simulink model "Boat_mode"  (R2019a)
settings: Solver=VariableStepAuto  StartTime=0.0  StopTime=3000  RelTol=1e-3
InitFcn:
  | w = 0.3;
  | boat_m = 600;
  | boat_m_x = 50;
  | boat_m_y = 100;
  | 
  | boat_I = 6000000;
  | boat_Iz = 10;
  | 
  | propeller_diameter = 1;
  | wake_friction=0.3;
  | 
  | c_r_front = 0.31;
  | c_r_side = 2;
  | thrust_deduction = 0.3;
  | 
  | rho = 1;
  | 
  | boat_area_front = 20;
  | boat_area_side = 90;
  | boat_l = 15;
  | boat_b = 6;
  | 
  | rudder_area = 10;
  | aspect_ratio = 2;
  | a = 4.252;
  | b = 0.262;
  | 
  | plot =20000;
libraries: simulink x7, simulink_extras x3
settings Model: Creator=nicos  LastModifiedBy=nicos
settings DataIOCC: SaveState=on

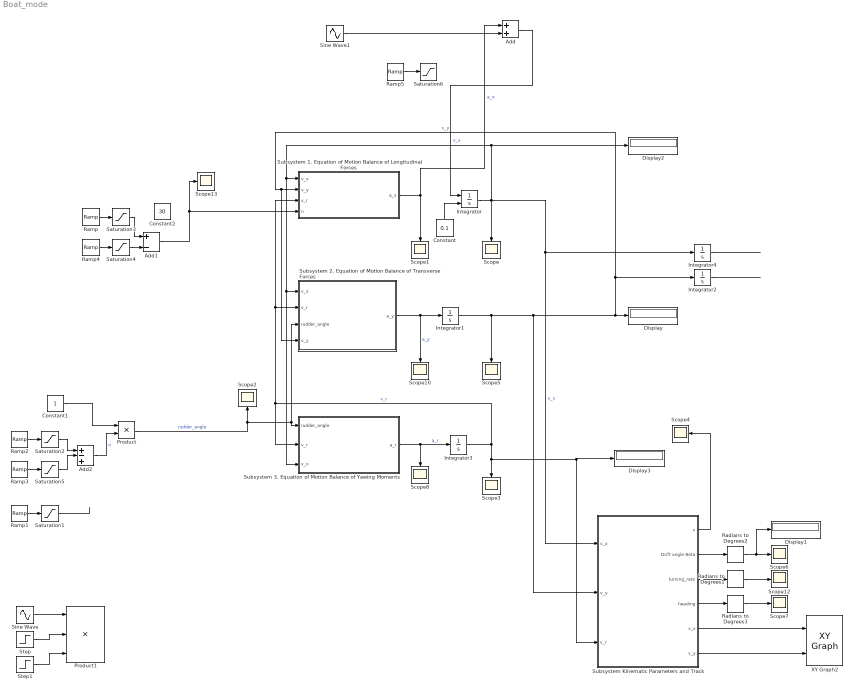
== system Boat_mode ==
  Add : Sum
  Add1 : Sum  Inputs=+-
  Add2 : Sum  Inputs=+-+
  Constant : Constant  Value=0.1
  Constant1 : Constant
  Constant2 : Constant  Value=30
  Display{,1..3} (4 alike) : Display
  Integrator : Integrator  InitialConditionSource=external  LimitOutput=on  LowerSaturationLimit=0
  Integrator{1..4} (4 alike) : Integrator
  Product : Product
  Product1 : Product  Inputs=3
  Radians to Degrees1 : simulink_extras/Transformations/Radians to Degrees
  Radians to Degrees2 : simulink_extras/Transformations/Radians to Degrees
  Radians to Degrees3 : simulink_extras/Transformations/Radians to Degrees
  Ramp : simulink/Sources/Ramp  slope=2  start=50  InitialOutput=0
  Ramp1 : simulink/Sources/Ramp  slope=0.01  start=1500  InitialOutput=0
  Ramp2 : simulink/Sources/Ramp  slope=0.01  start=500  InitialOutput=0
  Ramp3 : simulink/Sources/Ramp  slope=0.01  start=1000  InitialOutput=0
  Ramp4 : simulink/Sources/Ramp  slope=0.1  start=1300  InitialOutput=0
  Ramp5 : simulink/Sources/Ramp  slope=0.1  start=500  InitialOutput=0
  Saturation1 : Saturate  UpperLimit=pi/4  LowerLimit=0
  Saturation2 : Saturate  UpperLimit=pi/4  LowerLimit=0
  Saturation3 : Saturate  UpperLimit=20  LowerLimit=0
  Saturation4 : Saturate  UpperLimit=20  LowerLimit=0
  Saturation5 : Saturate  UpperLimit=pi/2  LowerLimit=0
  Saturation6 : Saturate  UpperLimit=1  LowerLimit=0
  Scope{,1..8,10,12..13} (12 alike) : Scope
  Sine Wave : Sin  Amplitude=pi/4  Frequency=0.01  SampleTime=0
  Sine Wave1 : Sin  Amplitude=0  Frequency=0.005  SampleTime=0
  Step : Step  Time=0  SampleTime=0
  Step1 : Step  Time=2000  Before=1  After=0  SampleTime=0
  Subsystem Kinematic Parameters and Track : Subsystem
  Subsystem 1. Equation of Motion Balance of Longitudinal Forces : Subsystem
  Subsystem 2. Equation of Motion Balance of Transverse Forces : Subsystem
  Subsystem 3. Equation of Motion Balance of Yawing Moments : Subsystem
  XY Graph2 : simulink/Sinks/XY Graph  xmin=-plot  xmax=plot  ymin=-plot  ymax=plot  st=-1
  wires:
  Subsystem 1. Equation of Motion Balance of Longitudinal Forces/1(a_x) -> Add/1, Scope1/1  "a_x"
  Constant/1 -> Integrator/2
  Integrator/1 -> Subsystem 2. Equation of Motion Balance of Transverse Forces/1(v_x), Subsystem 3. Equation of Motion Balance of Yawing Moments/3(v_x), Subsystem 1. Equation of Motion Balance of Longitudinal Forces/1(v_x), Display2/1, Integrator4/1, Subsystem Kinematic Parameters and Track/1(v_x), Scope/1  "v_x"
  Subsystem 3. Equation of Motion Balance of Yawing Moments/1(a_r) -> Integrator3/1, Scope8/1  "a_r"
  Subsystem 2. Equation of Motion Balance of Transverse Forces/1(a_y) -> Integrator1/1, Scope10/1  "a_y"
  Subsystem Kinematic Parameters and Track/1(v) -> Scope4/1
  Subsystem Kinematic Parameters and Track/5(s_x) -> XY Graph2/1
  Subsystem Kinematic Parameters and Track/6(s_y) -> XY Graph2/2
  Ramp4/1 -> Saturation4/1
  Saturation3/1 -> Add1/1
  Saturation4/1 -> Add1/2
  Ramp/1 -> Saturation3/1
  Subsystem Kinematic Parameters and Track/2(Drift angle Beta) -> Radians to Degrees2/1
  Subsystem Kinematic Parameters and Track/3(turning_rate) -> Radians to Degrees1/1
  Radians to Degrees1/1 -> Scope12/1
  Radians to Degrees2/1 -> Display1/1, Scope6/1
  Subsystem Kinematic Parameters and Track/4(heading) -> Radians to Degrees3/1
  Radians to Degrees3/1 -> Scope7/1
  Integrator3/1 -> Subsystem 2. Equation of Motion Balance of Transverse Forces/2(v_r), Subsystem 1. Equation of Motion Balance of Longitudinal Forces/3(v_r), Subsystem 3. Equation of Motion Balance of Yawing Moments/2(v_r), Display3/1, Subsystem Kinematic Parameters and Track/3(v_r), Scope3/1  "v_r"
  Product/1 -> Scope2/1, Subsystem 2. Equation of Motion Balance of Transverse Forces/3(rudder_angle), Subsystem 3. Equation of Motion Balance of Yawing Moments/1(rudder_angle)  "rudder_angle"
  Constant1/1 -> Product/1
  Integrator4/1 -> ?
  Integrator2/1 -> ?
  Saturation2/1 -> Add2/1
  Ramp3/1 -> Saturation5/1
  Saturation5/1 -> Add2/2
  Ramp2/1 -> Saturation2/1
  Add2/1 -> Product/2  "n"
  Add1/1 -> Subsystem 1. Equation of Motion Balance of Longitudinal Forces/4(n), Scope13/1
  Ramp1/1 -> Saturation1/1
  Saturation1/1 -> ?
  Sine Wave/1 -> Product1/1
  Step/1 -> Product1/2
  Step1/1 -> Product1/3
  Integrator1/1 -> Scope5/1, Subsystem Kinematic Parameters and Track/2(v_y), Display/1, Integrator2/1, Subsystem 2. Equation of Motion Balance of Transverse Forces/4(v_y), Subsystem 1. Equation of Motion Balance of Longitudinal Forces/2(v_y)  "v_y"
  Sine Wave1/1 -> Add/2
  Ramp5/1 -> Saturation6/1
  Add/1 -> Integrator/1  "v_x"

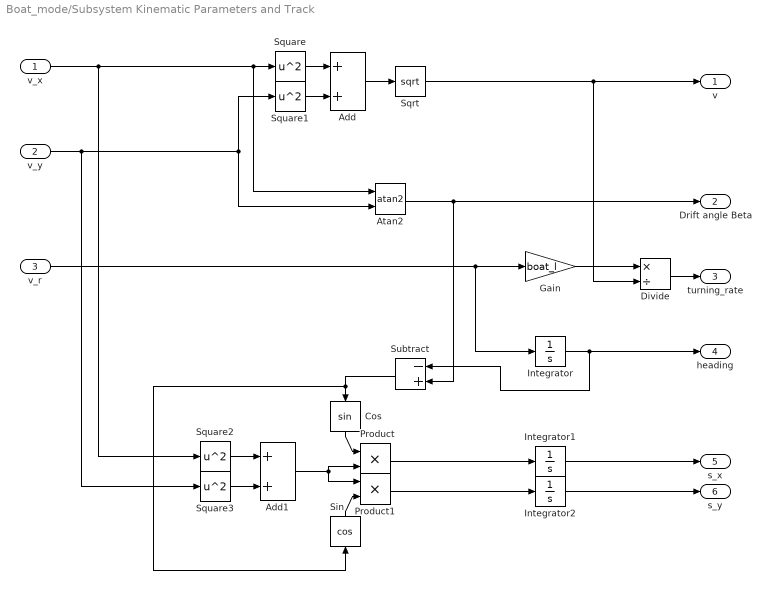
== system Boat_mode/Subsystem Kinematic Parameters and Track ==
  v_x : Inport
  v_y : Inport  Port=2
  v_r : Inport  Port=3
  Add : Sum
  Add1 : Sum
  Atan2 : Trigonometry  Operator=atan2
  Cos : Trigonometry
  Divide : Product  Inputs=*/
  Gain : Gain  Gain=boat_l
  Integrator : Integrator
  Integrator1 : Integrator
  Integrator2 : Integrator
  Product : Product
  Product1 : Product
  Sin : Trigonometry  Operator=cos
  Sqrt : Sqrt  SaturateOnIntegerOverflow=on
  Square{,1..3} (4 alike) : Math  Operator=square  SaturateOnIntegerOverflow=on
  Subtract : Sum  Inputs=-+
  v : Outport
  Drift angle Beta : Outport  Port=2
  turning_rate : Outport  Port=3
  heading : Outport  Port=4
  s_x : Outport  Port=5
  s_y : Outport  Port=6
  wires:
  v_x/1 -> Square2/1, Atan2/1, Square/1
  v_y/1 -> Square3/1, Atan2/2, Square1/1
  Square/1 -> Add/1
  Square1/1 -> Add/2
  Add/1 -> Sqrt/1
  Sqrt/1 -> v/1, Divide/2
  Gain/1 -> Divide/1
  Divide/1 -> turning_rate/1
  v_r/1 -> Integrator/1, Gain/1
  Integrator/1 -> Subtract/1, heading/1
  Integrator1/1 -> s_x/1
  Integrator2/1 -> s_y/1
  Atan2/1 -> Subtract/2, Drift angle Beta/1
  Square2/1 -> Add1/1
  Square3/1 -> Add1/2
  Add1/1 -> Product1/1, Product/2
  Subtract/1 -> Sin/1, Cos/1
  Cos/1 -> Product/1
  Product/1 -> Integrator1/1
  Product1/1 -> Integrator2/1
  Sin/1 -> Product1/2

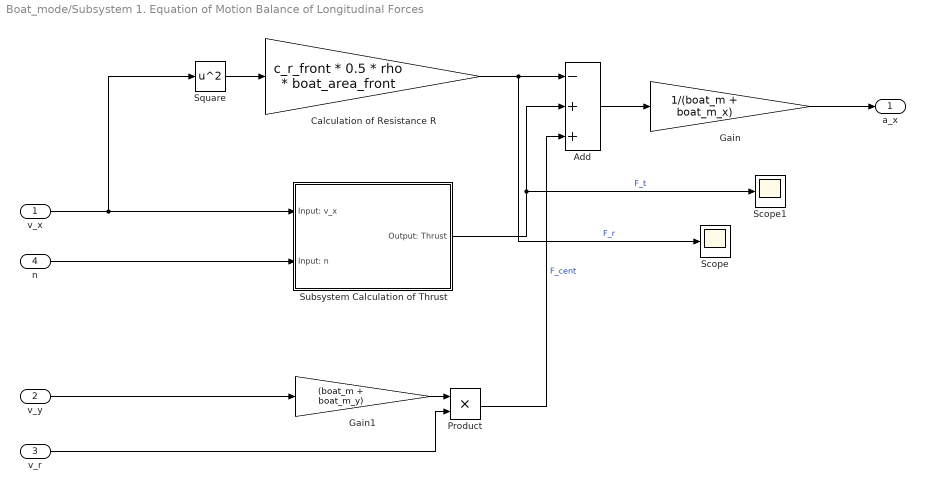
== system Boat_mode/Subsystem 1. Equation of Motion Balance of Longitudinal Forces ==
  v_x : Inport
  v_y : Inport  Port=2
  v_r : Inport  Port=3
  n : Inport  Port=4
  Add : Sum  Inputs=-++
  Calculation of Resistance R : Gain  Gain=c_r_front * 0.5 * rho * boat_area_front
  Gain : Gain  Gain=1/(boat_m + boat_m_x)
  Gain1 : Gain  Gain=(boat_m + boat_m_y)
  Product : Product
  Scope : Scope
  Scope1 : Scope
  Square : Math  Operator=square  SaturateOnIntegerOverflow=on
  Subsystem Calculation of Thrust : Subsystem
  a_x : Outport
  wires:
  v_x/1 -> Square/1, Subsystem Calculation of Thrust/1(Input: v_x)
  n/1 -> Subsystem Calculation of Thrust/2(Input: n)
  Square/1 -> Calculation of Resistance R/1
  Calculation of Resistance R/1 -> Scope/1, Add/1  "F_r"
  Subsystem Calculation of Thrust/1(Output: Thrust) -> Scope1/1, Add/2  "F_t"
  Add/1 -> Gain/1
  Gain/1 -> a_x/1
  v_y/1 -> Gain1/1
  Gain1/1 -> Product/1
  v_r/1 -> Product/2
  Product/1 -> Add/3  "F_cent"

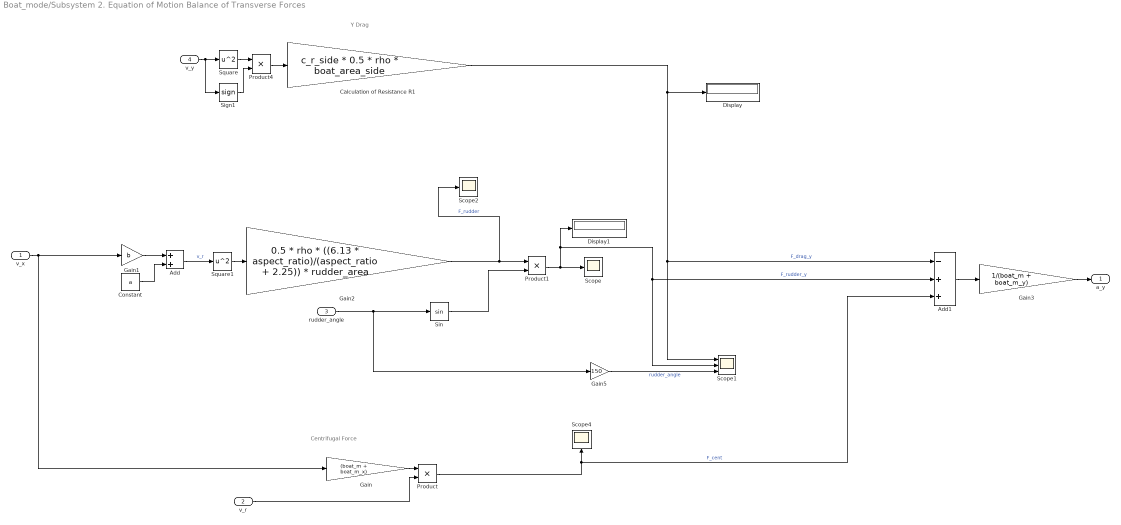
== system Boat_mode/Subsystem 2. Equation of Motion Balance of Transverse Forces ==
  note: Y Drag
  note: Centrifugal Force
  v_x : Inport
  v_r : Inport  Port=2
  rudder_angle : Inport  Port=3
  v_y : Inport  Port=4
  Add : Sum
  Add1 : Sum  Inputs=-++
  Calculation of Resistance R1 : Gain  Gain=c_r_side * 0.5 * rho * boat_area_side
  Constant : Constant  Value=a
  Display : Display
  Display1 : Display
  Gain : Gain  Gain=(boat_m + boat_m_x)
  Gain1 : Gain  Gain=b
  Gain2 : Gain  Gain=0.5 * rho * ((6.13 * aspect_ratio)/(aspect_ratio + 2.25)) * rudder_area
  Gain3 : Gain  Gain=1/(boat_m + boat_m_y)
  Gain5 : Gain  Gain=150
  Product : Product
  Product1 : Product
  Product4 : Product
  Scope : Scope
  Scope1 : Scope  NumInputPorts=3
  Scope2 : Scope
  Scope4 : Scope
  Sign1 : Signum
  Sin : Trigonometry
  Square : Math  Operator=square  SaturateOnIntegerOverflow=on
  Square1 : Math  Operator=square  SaturateOnIntegerOverflow=on
  a_y : Outport
  wires:
  Gain/1 -> Product/1
  v_r/1 -> Product/2
  Gain1/1 -> Add/1
  Constant/1 -> Add/2
  v_x/1 -> Gain1/1, Gain/1
  Square1/1 -> Gain2/1
  Add1/1 -> Gain3/1
  Square/1 -> Product4/1
  v_y/1 -> Sign1/1, Square/1
  Gain2/1 -> Product1/1, Scope2/1  "F_rudder"
  Add/1 -> Square1/1  "v_r"
  Sin/1 -> Product1/2
  Product/1 -> Add1/3, Scope4/1  "F_cent"
  rudder_angle/1 -> Sin/1, Gain5/1
  Product1/1 -> Display1/1, Add1/2, Scope1/2, Scope/1  "F_rudder_y"
  Gain5/1 -> Scope1/3  "rudder_angle"
  Gain3/1 -> a_y/1
  Calculation of Resistance R1/1 -> Scope1/1, Add1/1, Display/1  "F_drag_y"
  Product4/1 -> Calculation of Resistance R1/1
  Sign1/1 -> Product4/2

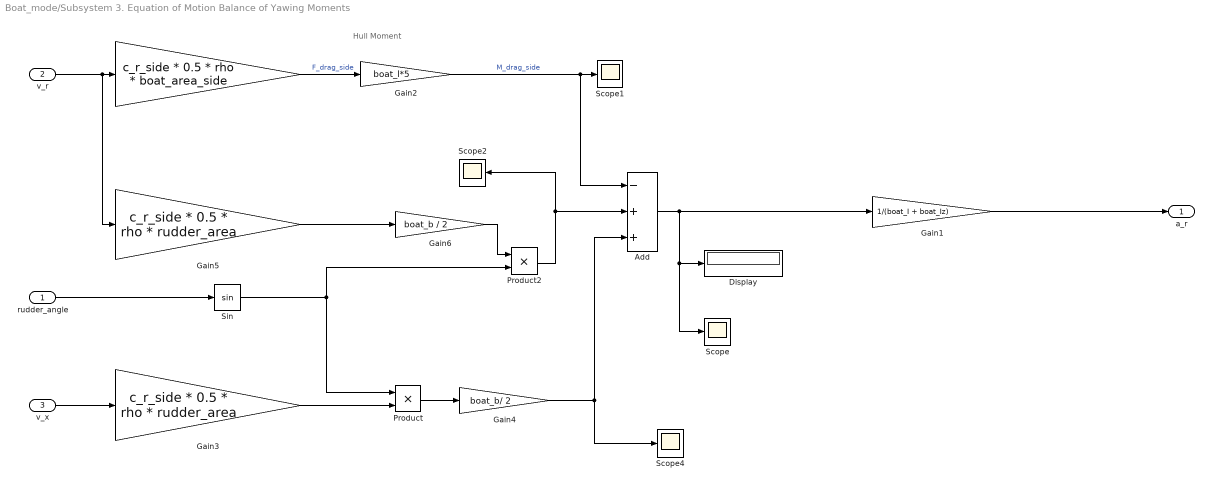
== system Boat_mode/Subsystem 3. Equation of Motion Balance of Yawing Moments ==
  note: Hull Moment
  rudder_angle : Inport
  v_r : Inport  Port=2
  v_x : Inport  Port=3
  " " : Gain  Gain=c_r_side * 0.5 * rho * boat_area_side
  Add : Sum  Inputs=-++
  Display : Display
  Gain1 : Gain  Gain=1/(boat_I + boat_Iz)
  Gain2 : Gain  Gain=boat_l*5
  Gain3 : Gain  Gain=c_r_side * 0.5 * rho * rudder_area
  Gain4 : Gain  Gain=boat_b/ 2
  Gain5 : Gain  Gain=c_r_side * 0.5 * rho * rudder_area
  Gain6 : Gain  Gain=boat_b / 2
  Product : Product
  Product2 : Product
  Scope{,1..2,4} (4 alike) : Scope
  Sin : Trigonometry
  a_r : Outport
  wires:
  " "/1 -> Gain2/1  "F_drag_side"
  Add/1 -> Scope/1, Display/1, Gain1/1
  Gain1/1 -> a_r/1
  Gain2/1 -> Add/1, Scope1/1  "M_drag_side"
  Gain6/1 -> Product2/1
  Gain5/1 -> Gain6/1
  Sin/1 -> Product2/2, Product/1
  rudder_angle/1 -> Sin/1
  v_r/1 -> Gain5/1, " "/1
  Gain3/1 -> Product/2
  Product/1 -> Gain4/1
  Gain4/1 -> Add/3, Scope4/1
  v_x/1 -> Gain3/1
  Product2/1 -> Scope2/1, Add/2

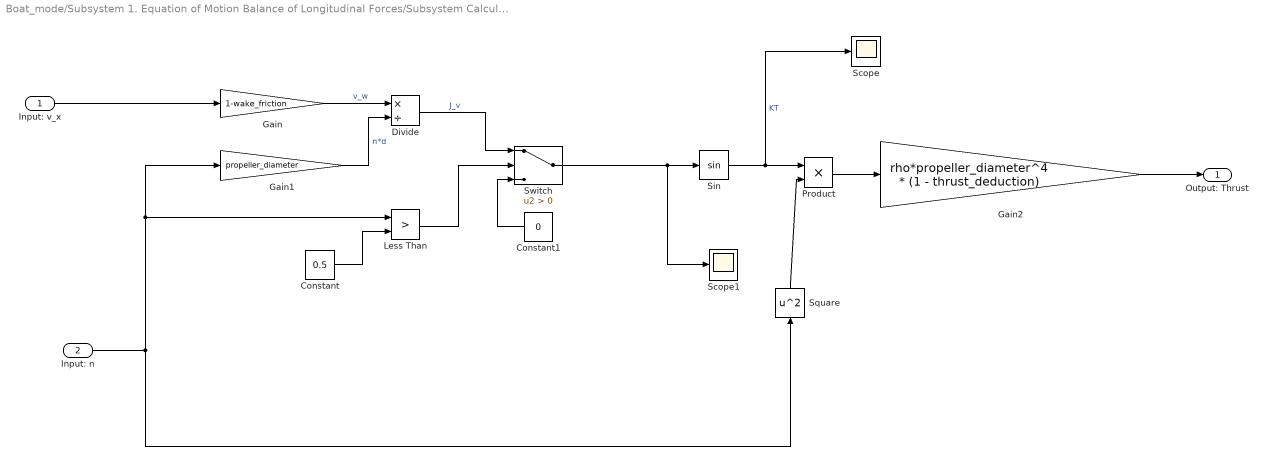
== system Boat_mode/Subsystem 1. Equation of Motion Balance of Longitudinal Forces/Subsystem Calculation of Thrust ==
  Input: v_x : Inport
  Input: n : Inport  Port=2
  Constant : Constant  Value=0.5
  Constant1 : Constant  Value=0
  Divide : Product  Inputs=*/
  Gain : Gain  Gain=1-wake_friction
  Gain1 : Gain  Gain=propeller_diameter
  Gain2 : Gain  Gain=rho*propeller_diameter^4 * (1 - thrust_deduction)
  Less Than : RelationalOperator  Operator=>  OutDataTypeStr=boolean  RndMeth=Simplest
  Product : Product
  Scope : Scope
  Scope1 : Scope
  Sin : Trigonometry
  Square : Math  Operator=square  SaturateOnIntegerOverflow=on
  Switch : Switch  Criteria=u2 > Threshold
  Output: Thrust : Outport
  wires:
  Input: n/1 -> Gain1/1, Less Than/1, Square/1
  Gain/1 -> Divide/1  "v_w"
  Gain1/1 -> Divide/2  "n*d"
  Divide/1 -> Switch/1  "J_v"
  Sin/1 -> Scope/1, Product/1  "KT"
  Gain2/1 -> Output: Thrust/1
  Square/1 -> Product/2
  Product/1 -> Gain2/1
  Constant1/1 -> Switch/3
  Less Than/1 -> Switch/2
  Constant/1 -> Less Than/2
  Switch/1 -> Scope1/1, Sin/1
  Input: v_x/1 -> Gain/1
